simulink model "AOO"  (R2023a)
settings: Solver=FixedStepAuto  StartTime=0.0  StopTime=10.0  FixedStep=1e-3  RelTol=1e-3  EnableMultiTasking=on
settings Model: ExtModeTrigDuration=5  Creator=tstic  LastModifiedBy=emcan
settings OptimizationCC: EnhancedBackFolding=on  PassReuseOutputArgsAs=Individual arguments  ZeroExternalMemoryAtStartup=off  ZeroInternalMemoryAtStartup=off  MaxStackSize=64  OptimizeBlockOrder=speed  DifferentSizesBufferReuse=on  OptimizationCustomize=off  EfficientTunableParamExpr=on
settings DebuggingCC: ParameterTunabilityLossMsg=error
settings HardwareCC: ProdBitPerPointer=32  ProdBitPerSizeT=32  ProdBitPerPtrDiffT=32  ProdLargestAtomicInteger=Long  ProdLargestAtomicFloat=Double  ProdWordSize=32  ProdHWDeviceType=ARM Compatible->ARM Cortex
settings SFSimCC: MATLABDynamicMemAlloc=off
settings RTWCC: Description=Embedded Coder  SystemTargetFile=ert.tlc  HardwareBoard=NXP FRDM-K64F  TLCOptions="-aInlineSetEventsForThisBaseRateFcn=TLC_FALSE -aSuppressMultiTaskScheduler=TLC_FALSE  -aRateBasedStepFcn=0"  TemplateMakefile=ert_default_tmf  Toolchain=GNU Tools for ARM Embedded Processors
settings CodeAppCC: ForceParamTrailComments=on  IgnoreCustomStorageClasses=off  OperatorAnnotations=on  SimulinkDataObjDesc=on  SFDataObjDesc=on  InsertBlockDesc=on
settings ERTTargetCC: ExtModeTransport=4  ExtModeMexFile=sendToCommService

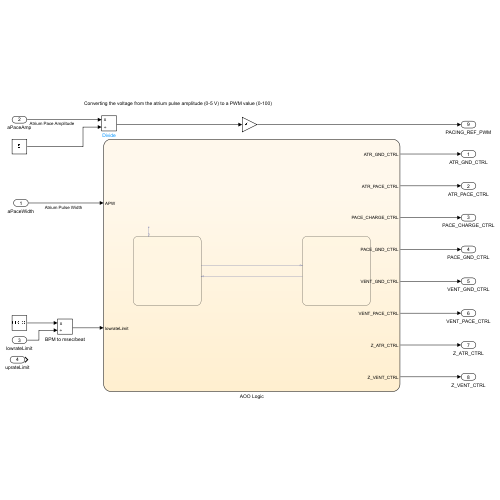
[thumbnail: Simulink's stored preview of the top-level diagram]
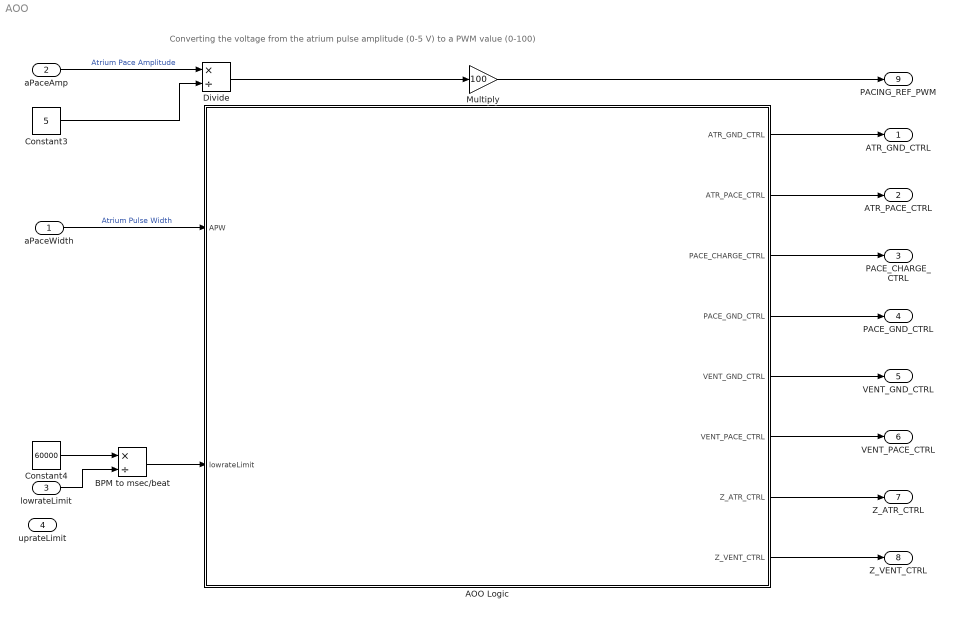
== system AOO ==
  note: Converting the voltage from the atrium pulse amplitude (0-5 V) to a PWM value (0-100)
  aPaceWidth : Inport
  aPaceAmp : Inport  Port=2
  lowrateLimit : Inport  Port=3
  uprateLimit : Inport  Port=4
  AOO Logic : Stateflow chart  TreatAsAtomicUnit=on
  BPM to msec/beat : Product  Inputs=*/
  Constant3 : Constant  Value=5
  Constant4 : Constant  Value=60000
  Divide : Product  Inputs=*/
  Multiply : Gain  Gain=100
  ATR_GND_CTRL : Outport
  ATR_PACE_CTRL : Outport  Port=2
  PACE_CHARGE_CTRL : Outport  Port=3
  PACE_GND_CTRL : Outport  Port=4
  VENT_GND_CTRL : Outport  Port=5
  VENT_PACE_CTRL : Outport  Port=6
  Z_ATR_CTRL : Outport  Port=7
  Z_VENT_CTRL : Outport  Port=8
  PACING_REF_PWM : Outport  Port=9
  wires:
  Multiply/1 -> PACING_REF_PWM/1
  aPaceWidth/1 -> AOO Logic/1(APW)  "Atrium Pulse Width"
  Divide/1 -> Multiply/1
  lowrateLimit/1 -> BPM to msec/beat/2
  Constant4/1 -> BPM to msec/beat/1
  Constant3/1 -> Divide/2
  aPaceAmp/1 -> Divide/1  "Atrium Pace Amplitude"
  BPM to msec/beat/1 -> AOO Logic/2(lowrateLimit)
  AOO Logic/5(VENT_GND_CTRL) -> VENT_GND_CTRL/1
  AOO Logic/1(ATR_GND_CTRL) -> ATR_GND_CTRL/1
  AOO Logic/6(VENT_PACE_CTRL) -> VENT_PACE_CTRL/1
  AOO Logic/2(ATR_PACE_CTRL) -> ATR_PACE_CTRL/1
  AOO Logic/7(Z_ATR_CTRL) -> Z_ATR_CTRL/1
  AOO Logic/3(PACE_CHARGE_CTRL) -> PACE_CHARGE_CTRL/1
  AOO Logic/8(Z_VENT_CTRL) -> Z_VENT_CTRL/1
  AOO Logic/4(PACE_GND_CTRL) -> PACE_GND_CTRL/1

== stateflow chart AOO/AOO Logic ==
  state ChargeDischargeAtrium
    entry:
    PACE_GND_CTRL = 1;
    ATR_PACE_CTRL = 0;
    Z_ATR_CTRL = 0;
    Z_VENT_CTRL = 0;
    VENT_PACE_CTRL = 0;
    VENT_GND_CTRL = 0;
    ATR_GND_CTRL = 1;
    during:
    PACE_CHARGE_CTRL = 1;
  state PaceAtrium
    entry:
    PACE_CHARGE_CTRL = 0;
    PACE_GND_CTRL = 1;
    VENT_PACE_CTRL = 0;
    VENT_GND_CTRL = 0;
    Z_VENT_CTRL = 0;
    Z_ATR_CTRL = 0;
    ATR_GND_CTRL = 0;
    ATR_PACE_CTRL = 1;
  note: Pace the atrium at the rate of the lowrateLimit
  note: Pace the atrium for the duration of the atrium pulse width
  (default) -> ChargeDischargeAtrium
  ChargeDischargeAtrium -> PaceAtrium : after(lowrateLimit - APW, msec)
  PaceAtrium -> ChargeDischargeAtrium : after(APW, msec)
  data: ATR_GND_CTRL output; ATR_PACE_CTRL output; PACE_CHARGE_CTRL output; PACE_GND_CTRL output; VENT_GND_CTRL output; VENT_PACE_CTRL output; Z_ATR_CTRL output; Z_VENT_CTRL output; APW input double =1; lowrateLimit input
